simulink model "carSim"  (R2022b)
settings: Solver=VariableStepAuto  StartTime=0.0  StopTime=10.0  RelTol=1e-3
values from neighbouring files (symbols this model uses):
  ws = 10    [sim_init.m]
  wt = 1    [sim_init.m]
  zetas = 0.7    [sim_init.m]
  zetat = 0.7    [sim_init.m]
settings Model: Creator=eduardorosado  LastModifiedBy=eduardorosado

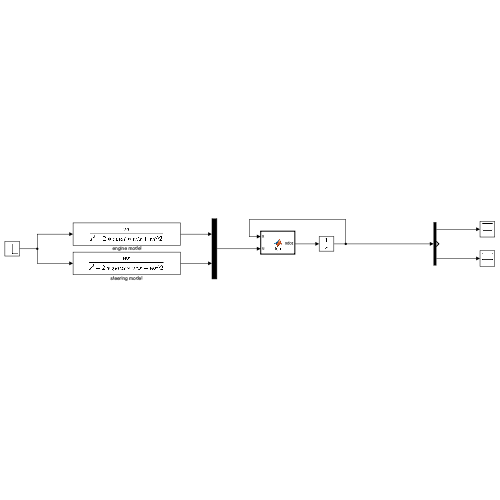
[thumbnail: Simulink's stored preview of the top-level diagram]
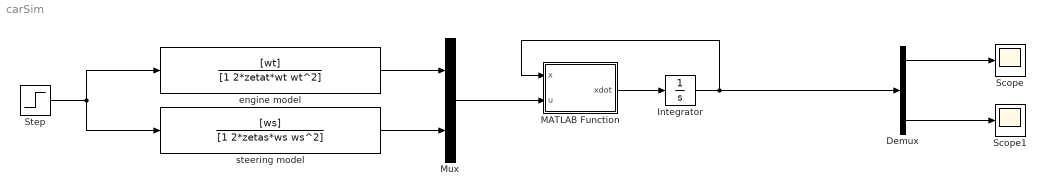
== system carSim ==
  " engine model" : TransferFcn  Numerator=[wt]  Denominator=[1 2*zetat*wt wt^2]
  Demux : Demux  Outputs=3
  Integrator : Integrator  InitialCondition=[0;0;0]
  MATLAB Function : MATLAB Function  TreatAsAtomicUnit=on
  Mux : Mux  Inputs=2
  Scope : Scope
  Scope1 : Scope
  Step : Step  Before=1  After=0  SampleTime=0
  steering model : TransferFcn  Numerator=[ws]  Denominator=[1 2*zetas*ws ws^2]
  wires:
  MATLAB Function/1(xdot) -> Integrator/1
  Integrator/1 -> Demux/1, MATLAB Function/1(x)
  Demux/1 -> Scope/1
  Demux/3 -> Scope1/1
  Step/1 -> " engine model"/1, steering model/1
  " engine model"/1 -> Mux/1
  steering model/1 -> Mux/2
  Mux/1 -> MATLAB Function/2(u)

== matlab function carSim/MATLAB Function ==
  data: x input; u input; xdot output
function xdot = fcn(x, u)

% sim setup

Iw = 3;
Ic = 30;
m = 80;
r = 3;
R = 15;
wheel_damp = 1;
turn_damp = 1;

wdot0 = u(1);
psi0 = u(2);


A = [0 1 0; 0 -wheel_damp 0; 0 0 -turn_damp];
B = [0 0; r*Iw/(m*r) 0; Iw*R*psi0/Ic Iw*R*wdot0/Ic];


xdot = A*x + B*u;
